simulink model "Scenario_2_v2"  (R2020b)
settings: Solver=ode1  StartTime=0.0  StopTime=10  FixedStep=Ts  MaxStep=Ts*2  MinStep=Ts/5  RelTol=1e-3
values from neighbouring files (symbols this model uses):
  c0 = c0_zeb    (= 6.57988e-09)    [Scenario_17_parameters_v2.m]    (also in Scenario_1_parameters_v2.m; Scenario_2_parameters_v2.m; Scenario_3_parameters_v2.m)
  c1 = c1_zeb    (= 9.15905e-09)    [Scenario_17_parameters_v2.m]    (also in Scenario_1_parameters_v2.m; Scenario_2_parameters_v2.m; Scenario_3_parameters_v2.m)
  fg = 50    [Scenario_17_parameters_v2.m]    (also in Scenario_1_parameters_v2.m; Scenario_2_parameters_v2.m; Scenario_3_parameters_v2.m)
  G1gen = 0.4692    [Scenario_17_parameters_v2.m]    (also in Scenario_1_parameters_v2.m = 0.1; Scenario_2_parameters_v2.m = 0.298581; Scenario_3_parameters_v2.m = 0.65)
  G2gen = 0.80    (= 0.8)    [Scenario_1_parameters_v2.m]    (also in Scenario_2_parameters_v2.m = 0.7; Scenario_3_parameters_v2.m = 0.4)
  G3gen = 0.85    [Scenario_1_parameters_v2.m]    (also in Scenario_2_parameters_v2.m = 0.9; Scenario_3_parameters_v2.m = 0.6)
  G4sgen = 0.8186    [Scenario_2_parameters_v2.m]
  G5gen = 0.75    [Scenario_17_parameters_v2.m]    (also in Scenario_1_parameters_v2.m = 0.8; Scenario_2_parameters_v2.m = 0.8; Scenario_3_parameters_v2.m = 0.705)
  G6gen = 0.90    (= 0.9)    [Scenario_17_parameters_v2.m]    (also in Scenario_1_parameters_v2.m; Scenario_2_parameters_v2.m = 0.81797; Scenario_3_parameters_v2.m = 0.45)
  G6sgen = 0.7    [Scenario_2_parameters_v2.m]
  G7gen = 0.20    (= 0.2)    [Scenario_17_parameters_v2.m]    (also in Scenario_1_parameters_v2.m = 0.5227; Scenario_2_parameters_v2.m = 0.5098; Scenario_3_parameters_v2.m = 0.4)
  Iovc = 1.2    [Scenario_17_parameters_v2.m]    (also in Scenario_1_parameters_v2.m; Scenario_2_parameters_v2.m; Scenario_3_parameters_v2.m)
  l0 = l0_zeb    (= 0.00368)    [Scenario_17_parameters_v2.m]    (also in Scenario_1_parameters_v2.m; Scenario_2_parameters_v2.m; Scenario_3_parameters_v2.m)
  l1 = l1_zeb    (= 0.00128)    [Scenario_17_parameters_v2.m]    (also in Scenario_1_parameters_v2.m; Scenario_2_parameters_v2.m; Scenario_3_parameters_v2.m)
  L3dem = 0.30    (= 0.3)    [Scenario_17_parameters_v2.m]    (also in Scenario_1_parameters_v2.m = 0.1; Scenario_2_parameters_v2.m = 0.1; Scenario_3_parameters_v2.m = 0.2)
  L4dem = 0.30    (= 0.3)    [Scenario_1_parameters_v2.m]    (also in Scenario_2_parameters_v2.m)
  L5dem = 0.25    [Scenario_17_parameters_v2.m]    (also in Scenario_1_parameters_v2.m = 0.35; Scenario_2_parameters_v2.m = 0.35; Scenario_3_parameters_v2.m = 0.1)
  L6dem = 0.15    [Scenario_1_parameters_v2.m]    (also in Scenario_2_parameters_v2.m; Scenario_3_parameters_v2.m = 0.1)
  L7dem = 0.10    (= 0.1)    [Scenario_1_parameters_v2.m]    (also in Scenario_2_parameters_v2.m; Scenario_3_parameters_v2.m = 0.2)
  Pr = Sr*PF    (= 1600500000)    [Scenario_17_parameters_v2.m]    (also in Scenario_1_parameters_v2.m = 1472500000; Scenario_2_parameters_v2.m = 1805000000; Scenario_3_parameters_v2.m = 12740000000)
  Qr = sqrt(Sr^2 - Pr^2)    [Scenario_17_parameters_v2.m]    (also in Scenario_1_parameters_v2.m; Scenario_2_parameters_v2.m; Scenario_3_parameters_v2.m)
  r0 = r0_zeb    (= 0.39362)    [Scenario_17_parameters_v2.m]    (also in Scenario_1_parameters_v2.m; Scenario_2_parameters_v2.m; Scenario_3_parameters_v2.m)
  r1 = r1_zeb    (= 0.06862)    [Scenario_17_parameters_v2.m]    (also in Scenario_1_parameters_v2.m; Scenario_2_parameters_v2.m; Scenario_3_parameters_v2.m)
  Rtpu = Xtpu/40    (= 0.0025)    [Scenario_17_parameters_v2.m]    (also in Scenario_1_parameters_v2.m = 0.00375; Scenario_2_parameters_v2.m = 0.00375; Scenario_3_parameters_v2.m)
  S1non = 700e6    (= 700000000)    [Scenario_17_parameters_v2.m]    (also in Scenario_1_parameters_v2.m = 400000000; Scenario_2_parameters_v2.m = 400000000; Scenario_3_parameters_v2.m = 1000000000)
  S2non = 300e6    (= 300000000)    [Scenario_1_parameters_v2.m]    (also in Scenario_2_parameters_v2.m; Scenario_3_parameters_v2.m = 3000000000)
  S3non = 200e6    (= 200000000)    [Scenario_1_parameters_v2.m]    (also in Scenario_2_parameters_v2.m; Scenario_3_parameters_v2.m = 1000000000)
  S4snon = 200e6    (= 200000000)    [Scenario_2_parameters_v2.m]
  S5non = 400e6    (= 400000000)    [Scenario_17_parameters_v2.m]    (also in Scenario_1_parameters_v2.m = 500000000; Scenario_2_parameters_v2.m = 500000000; Scenario_3_parameters_v2.m = 2000000000)
  S6non = 150e6    (= 150000000)    [Scenario_17_parameters_v2.m]    (also in Scenario_1_parameters_v2.m = 400000000; Scenario_2_parameters_v2.m = 400000000; Scenario_3_parameters_v2.m = 3000000000)
  S6snon = 200e6    (= 200000000)    [Scenario_2_parameters_v2.m]
  S7non = 1500e6    (= 1500000000)    [Scenario_17_parameters_v2.m]    (also in Scenario_1_parameters_v2.m = 200000000; Scenario_2_parameters_v2.m = 200000000; Scenario_3_parameters_v2.m = 4000000000)
  tonvsc = 0    [Scenario_17_parameters_v2.m]    (also in Scenario_1_parameters_v2.m; Scenario_2_parameters_v2.m; Scenario_3_parameters_v2.m = 0.0001)
  Ts = 50e-6    (= 5e-05)    [Scenario_17_parameters_v2.m]    (also in Scenario_1_parameters_v2.m = 0.0002; Scenario_2_parameters_v2.m = 2e-05; Scenario_3_parameters_v2.m = 0.0001)
  Vhv = 220e3    (= 220000)    [Scenario_17_parameters_v2.m]    (also in Scenario_1_parameters_v2.m; Scenario_2_parameters_v2.m; Scenario_3_parameters_v2.m)
  Vmv = 22e3    (= 22000)    [Scenario_17_parameters_v2.m]    (also in Scenario_1_parameters_v2.m; Scenario_2_parameters_v2.m; Scenario_3_parameters_v2.m)
  w_pll = 2*pi*80    (= 502.654824574)    [Scenario_17_parameters_v2.m]    (also in Scenario_1_parameters_v2.m; Scenario_2_parameters_v2.m; Scenario_3_parameters_v2.m)
  wc1 = wsw1/10    (= 848.230016469)    [Scenario_17_parameters_v2.m]    (also in Scenario_1_parameters_v2.m; Scenario_2_parameters_v2.m; Scenario_3_parameters_v2.m)
  wdc1 = wc1/10    (= 84.8230016469)    [Scenario_17_parameters_v2.m]    (also in Scenario_1_parameters_v2.m; Scenario_2_parameters_v2.m; Scenario_3_parameters_v2.m)
  wpq1 = wc1/10    (= 84.8230016469)    [Scenario_17_parameters_v2.m]    (also in Scenario_1_parameters_v2.m; Scenario_2_parameters_v2.m; Scenario_3_parameters_v2.m)
  wsw1 = ksw1*2*pi*fg    (= 8482.30016469)    [Scenario_17_parameters_v2.m]    (also in Scenario_1_parameters_v2.m; Scenario_2_parameters_v2.m; Scenario_3_parameters_v2.m)
  Xtpu = 0.10    (= 0.1)    [Scenario_17_parameters_v2.m]    (also in Scenario_1_parameters_v2.m = 0.15; Scenario_2_parameters_v2.m = 0.15; Scenario_3_parameters_v2.m)
undefined symbols (not defined in the file or in its folder): D11, Delta, Newton, Raphson
libraries: powerlib x214, simulink_extras x133, powerlib_meascontrol x102, pid_lib x48, simulink x32, eeTransforms x24, spsFirstOrderFilterLib x16, eePwmGeneratorTwoLevel x4
(part 18 of 19)

== system Scenario_2_v2/G6/VSC v2/VSC Control/Modulation/EMT Switching/Corrects delay1 ==
  Clock : Clock
  Filter delay : Constant  Commented=on  Value=tfilt
  Filter delay1 : Constant  Commented=on  Value=1/wsw1
  Gain : Gain  Gain=-2*pi*fg
  Memory : Memory
  Sum : Sum  Inputs=|+-
  Sum1 : Sum  Inputs=+++
  Sum2 : Sum  Inputs=|++
  Transformer connection : Constant  Value=pi/6
  dphi : Outport
  wires:
  Filter delay1/1 -> Sum1/1  "Tf"
  Filter delay/1 -> Sum1/3  "Tf"
  Sum/1 -> Sum1/2  "Ts"
  Clock/1 -> Memory/1, Sum/1
  Memory/1 -> Sum/2
  Sum1/1 -> Gain/1  "Td"
  Gain/1 -> Sum2/1
  Transformer connection/1 -> Sum2/2  "Tf"
  Sum2/1 -> dphi/1

== system Scenario_2_v2/G6/VSC v2/VSC Control/Modulation/Phasor I and Phasor PQ/Inverse Park Transform (Phasor) ==
  note: Transforming from real domain to complex domain
  note: In time domain, all variables are real.
      | In phasor domain, they are complex.
      | In phasor domain, what is seen as a variation in real domain is actually an angular displacement
      | As we know that the system is balanced, d and q have the same magnitude and are shifted 90 degrees
      | Thus, having the real parts and knowing that they are shifter 90 degrees, we can recover the complex part
  dq0 : Inport
  theta : Inport  Port=2
  Complex to Magnitude-Angle : ComplexToMagnitudeAngle  Commented=on
  Constant : Constant  Commented=on  Value=exp(-1i*2*pi/3)
  Constant1 : Constant  Commented=on  Value=exp(-1i*4*pi/3)
  Constant2 : Constant  Value=0
  Demux : Demux  Outputs=2
  Demux1 : Demux  Commented=on  Outputs=3
  Exp : Math  OutputSignalType=complex  SaturateOnIntegerOverflow=on
  Exp1 : Math  Commented=on  OutputSignalType=complex  SaturateOnIntegerOverflow=on
  First-Order Filter1 : spsFirstOrderFilterLib/First-Order Filter  Commented=on  FilterType=Lowpass  Tc=100e-6  Ts=0  Initialize=off  Vac_Init=[0, 0, 60]  Vdc_Init=0  PlotResponse=off  FreqRange="[0,  200,  1]"
  First-Order Filter2 : spsFirstOrderFilterLib/First-Order Filter  Commented=on  FilterType=Lowpass  Tc=100e-6  Ts=0  Initialize=off  Vac_Init=[0, 0, 60]  Vdc_Init=0  PlotResponse=off  FreqRange="[0,  200,  1]"
  Gain : Gain  Commented=on  Gain=exp(-1i*2*pi/3)
  Gain1 : Gain  Gain=1/2
  Gain2 : Gain  Gain=sqrt(3)
  Gain3 : Gain  Gain=1/2
  Gain4 : Gain  Gain=sqrt(3)
  Gain5 : Gain  Gain=1i
  Gain6 : Gain  Gain=-1
  Gain7 : Gain  Commented=on  Gain=1i
  Gain8 : Gain  Commented=on  Gain=exp(-1i*4*pi/3)
  Magnitude-Angle to Complex : MagnitudeAngleToComplex  Commented=on
  Mux : Mux  Commented=on  Inputs=3
  Mux2 : Mux  Inputs=3
  Product : Product
  Product1 : Product  Commented=on
  Real-Imag to Complex : RealImagToComplex
  Real-Imag to Complex1 : RealImagToComplex
  Sum : Sum  Inputs=|++
  Sum1 : Sum  Inputs=-|-
  Sum2 : Sum  Inputs=-|+
  Terminator : Terminator  Commented=on
  Terminator1 : Terminator  Commented=on
  abc : Outport  VectorParamsAs1DForOutWhenUnconnected=off
  wires:
  ? -> Demux1/1
  Demux1/3 -> Terminator1/1
  Magnitude-Angle to Complex/1 -> Gain/1, Mux/1, Gain8/1
  Gain/1 -> Mux/2
  Complex to Magnitude-Angle/1 -> First-Order Filter1/1
  Demux1/1 -> Complex to Magnitude-Angle/1
  Mux/1 -> ?
  Gain8/1 -> Mux/3
  Demux1/2 -> Terminator/1
  Complex to Magnitude-Angle/2 -> First-Order Filter2/1
  First-Order Filter2/1 -> Magnitude-Angle to Complex/2
  First-Order Filter1/1 -> Magnitude-Angle to Complex/1
  Sum/1 -> abc/1
  Constant2/1 -> [x0]
  Exp1/1 -> Product1/2
  Gain7/1 -> Exp1/1
  Gain6/1 -> Real-Imag to Complex1/2
  [xdr] -> Gain6/1
  [xqr] -> Real-Imag to Complex/2
  [xqr] -> Real-Imag to Complex1/1
  Real-Imag to Complex1/1 -> [xq]
  [xdr] -> Real-Imag to Complex/1
  Real-Imag to Complex/1 -> [xd]
  Gain3/1 -> Mux2/3
  Gain1/1 -> Mux2/2
  Sum2/1 -> Gain3/1
  [xd] -> Gain4/1
  [xq] -> Sum2/1
  Gain4/1 -> Sum2/2
  Gain2/1 -> Sum1/2
  [xd] -> Gain2/1
  [xq] -> Sum1/1
  Sum1/1 -> Gain1/1
  [xq] -> Mux2/1
  theta/1 -> Gain5/1
  Gain5/1 -> Exp/1
  Mux2/1 -> Product/1
  Exp/1 -> Product/2
  Product/1 -> Sum/1
  [x0] -> Sum/2
  Demux/2 -> [xqr]
  Demux/1 -> [xdr]
  dq0/1 -> Demux/1

== system Scenario_2_v2/G6/VSC v2/VSC Control/Modulation/Phasor I and Phasor PQ/Subsystem ==
  note: Symmetrical components to ABC
  012 : Inport
  Gain1 : Gain  Gain=[1 a a2]  SaturateOnIntegerOverflow=on  OutDataTypeStr=Inherit: Same as input  ParamDataTypeStr=Inherit: Same as input
  Gain2 : Gain  Gain=[1 a2 a]  SaturateOnIntegerOverflow=on  OutDataTypeStr=Inherit: Same as input  ParamDataTypeStr=Inherit: Same as input
  Mux : Mux  Inputs=3
  Sum : Sum  Inputs=1  InputSameDT=on  SaturateOnIntegerOverflow=on  OutDataTypeStr=Inherit: Same as first input
  Sum1 : Sum  Inputs=1  InputSameDT=on  SaturateOnIntegerOverflow=on  OutDataTypeStr=Inherit: Same as first input
  Sum2 : Sum  Inputs=1  InputSameDT=on  SaturateOnIntegerOverflow=on  OutDataTypeStr=Inherit: Same as first input
  abc : Outport
  wires:
  Mux/1 -> abc/1
  Sum2/1 -> Mux/1
  Sum/1 -> Mux/2
  Sum1/1 -> Mux/3
  Gain1/1 -> Sum1/1
  012/1 -> Gain2/1, Sum2/1, Gain1/1
  Gain2/1 -> Sum/1

== system Scenario_2_v2/G6/VSC v2/VSC Control/Modulation/Phasor Quasi-EMT/Corrects delay ==
  Clock : Clock
  Gain : Gain  Gain=(2*pi*fg)
  Memory : Memory
  Sum : Sum  Inputs=|+-
  Sum2 : Sum  Inputs=|++
  Transformer connection : Constant  Commented=on  Value=pi/6
  dphi : Outport
  wires:
  Clock/1 -> Memory/1, Sum/1
  Memory/1 -> Sum/2
  Sum/1 -> Gain/1  "Ts"
  Transformer connection/1 -> Sum2/2  "Tf"
  Gain/1 -> Sum2/1
  Sum2/1 -> dphi/1

== system Scenario_2_v2/G6/VSC v2/VSC Control/Modulation/Phasor Quasi-EMT/Corrects delay2 ==
  Clock : Clock
  Gain : Gain  Gain=(2*pi*fg)
  Memory : Memory
  Sum : Sum  Inputs=|+-
  Sum2 : Sum  Inputs=|++
  Transformer connection : Constant  Commented=on  Value=pi/6
  dphi : Outport
  wires:
  Clock/1 -> Memory/1, Sum/1
  Memory/1 -> Sum/2
  Sum/1 -> Gain/1  "Ts"
  Transformer connection/1 -> Sum2/2  "Tf"
  Gain/1 -> Sum2/1
  Sum2/1 -> dphi/1

== system Scenario_2_v2/G6/VSC v2/VSC Control/Modulation/Phasor Quasi-EMT/Inverse Park Transform (Phasor) ==
  note: In time domain, all variables are real.
      | In phasor domain, they are complex.
      | In phasor domain, what is seen as a variation in real domain is actually an angular displacement
      | As we know that the system is balanced, d and q have the same magnitude and are shifted 90 degrees
      | Thus, having the real parts and knowing that they are shifter 90 degrees, we can recover the complex part
  note: Transforming from real domain to complex domain
  dq0 : Inport
  theta : Inport  Port=2
  Complex to Magnitude-Angle : ComplexToMagnitudeAngle  Commented=on
  Constant : Constant  Commented=on  Value=exp(-1i*2*pi/3)
  Constant1 : Constant  Commented=on  Value=exp(-1i*4*pi/3)
  Constant2 : Constant  Value=0
  Demux : Demux  Outputs=2
  Demux1 : Demux  Commented=on  Outputs=3
  Exp : Math  OutputSignalType=complex  SaturateOnIntegerOverflow=on
  Exp1 : Math  Commented=on  OutputSignalType=complex  SaturateOnIntegerOverflow=on
  First-Order Filter1 : spsFirstOrderFilterLib/First-Order Filter  Commented=on  FilterType=Lowpass  Tc=100e-6  Ts=0  Initialize=off  Vac_Init=[0, 0, 60]  Vdc_Init=0  PlotResponse=off  FreqRange="[0,  200,  1]"
  First-Order Filter2 : spsFirstOrderFilterLib/First-Order Filter  Commented=on  FilterType=Lowpass  Tc=100e-6  Ts=0  Initialize=off  Vac_Init=[0, 0, 60]  Vdc_Init=0  PlotResponse=off  FreqRange="[0,  200,  1]"
  Gain : Gain  Commented=on  Gain=exp(-1i*2*pi/3)
  Gain1 : Gain  Gain=1/2
  Gain2 : Gain  Gain=sqrt(3)
  Gain3 : Gain  Gain=1/2
  Gain4 : Gain  Gain=sqrt(3)
  Gain5 : Gain  Gain=1i
  Gain6 : Gain  Gain=-1
  Gain7 : Gain  Commented=on  Gain=1i
  Gain8 : Gain  Commented=on  Gain=exp(-1i*4*pi/3)
  Magnitude-Angle to Complex : MagnitudeAngleToComplex  Commented=on
  Mux : Mux  Commented=on  Inputs=3
  Mux2 : Mux  Inputs=3
  Product : Product
  Product1 : Product  Commented=on
  Real-Imag to Complex : RealImagToComplex
  Real-Imag to Complex1 : RealImagToComplex
  Sum : Sum  Inputs=|++
  Sum1 : Sum  Inputs=-|-
  Sum2 : Sum  Inputs=-|+
  Terminator : Terminator  Commented=on
  Terminator1 : Terminator  Commented=on
  abc : Outport  VectorParamsAs1DForOutWhenUnconnected=off
  wires:
  dq0/1 -> Demux/1
  Demux/1 -> [xdr]
  Demux/2 -> [xqr]
  [x0] -> Sum/2
  Product/1 -> Sum/1
  Exp/1 -> Product/2
  Mux2/1 -> Product/1
  Gain5/1 -> Exp/1
  theta/1 -> Gain5/1
  [xq] -> Mux2/1
  Sum1/1 -> Gain1/1
  [xq] -> Sum1/1
  [xd] -> Gain2/1
  Gain2/1 -> Sum1/2
  Gain4/1 -> Sum2/2
  [xq] -> Sum2/1
  [xd] -> Gain4/1
  Sum2/1 -> Gain3/1
  Gain1/1 -> Mux2/2
  Gain3/1 -> Mux2/3
  Real-Imag to Complex/1 -> [xd]
  [xdr] -> Real-Imag to Complex/1
  Real-Imag to Complex1/1 -> [xq]
  [xqr] -> Real-Imag to Complex1/1
  [xqr] -> Real-Imag to Complex/2
  [xdr] -> Gain6/1
  Gain6/1 -> Real-Imag to Complex1/2
  Gain7/1 -> Exp1/1
  Exp1/1 -> Product1/2
  Constant2/1 -> [x0]
  Sum/1 -> abc/1
  First-Order Filter1/1 -> Magnitude-Angle to Complex/1
  First-Order Filter2/1 -> Magnitude-Angle to Complex/2
  Complex to Magnitude-Angle/2 -> First-Order Filter2/1
  Demux1/2 -> Terminator/1
  Gain8/1 -> Mux/3
  Mux/1 -> ?
  Demux1/1 -> Complex to Magnitude-Angle/1
  Complex to Magnitude-Angle/1 -> First-Order Filter1/1
  Gain/1 -> Mux/2
  Magnitude-Angle to Complex/1 -> Gain8/1, Mux/1, Gain/1
  Demux1/3 -> Terminator1/1
  ? -> Demux1/1

== system Scenario_2_v2/G6/VSC v2/VSC Control/Modulation/Phasor Quasi-EMT/Subsystem ==
  note: Symmetrical components to ABC
  012 : Inport
  Gain1 : Gain  Gain=[1 a a2]  SaturateOnIntegerOverflow=on  OutDataTypeStr=Inherit: Same as input  ParamDataTypeStr=Inherit: Same as input
  Gain2 : Gain  Gain=[1 a2 a]  SaturateOnIntegerOverflow=on  OutDataTypeStr=Inherit: Same as input  ParamDataTypeStr=Inherit: Same as input
  Mux : Mux  Inputs=3
  Sum : Sum  Inputs=1  InputSameDT=on  SaturateOnIntegerOverflow=on  OutDataTypeStr=Inherit: Same as first input
  Sum1 : Sum  Inputs=1  InputSameDT=on  SaturateOnIntegerOverflow=on  OutDataTypeStr=Inherit: Same as first input
  Sum2 : Sum  Inputs=1  InputSameDT=on  SaturateOnIntegerOverflow=on  OutDataTypeStr=Inherit: Same as first input
  abc : Outport
  wires:
  Gain2/1 -> Sum/1
  012/1 -> Gain1/1, Sum2/1, Gain2/1
  Gain1/1 -> Sum1/1
  Sum1/1 -> Mux/3
  Sum/1 -> Mux/2
  Sum2/1 -> Mux/1
  Mux/1 -> abc/1

== system Scenario_2_v2/G6/VSC v2/VSC Control/Modulation/Phasor Quasi-EMT/V to I RL (+seq) ==
  note: d-q axis model of a 3-phase series R-L branch
  note: Using Laplace transform:
  note: Iq = (Vq1 - Vq2 - w*L*Id)/(R + s*L)
  note: Id = (Vd1 - Vd2 + w*L*Iq)/(R + s*L)
  note: V2
  note: ==========================================================================================
  note: V1
  note: Vq1 - Vq2 = [ R * Iq ] + [ L* w * Id ] + [ L * d/dt (Iq) ]
  note: where w = 2*pi*f
  note: I --->
  note: o--------| R |---| L |-------o
  note: Vd1 - Vd2 = [ R * Id ] - [ L* w * Iq ] + [ L * d/dt (Id) ]
  note: This subsystem converts the VSC output voltage in a current signal through an RL element
  Vdq1 : Inport
  Vdq2 : Inport  Port=2
  Cartesian to Polar : simulink_extras/Transformations/Cartesian to Polar
  Delay : Delay  DelayLength=1
  Demux : Demux  Outputs=2
  IC : InitialCondition  Value=Tcd
  IC1 : InitialCondition  Value=Tcq
  Mux : Mux  Inputs=2
  Polar to Cartesian : simulink_extras/Transformations/Polar to Cartesian
      settings: SourceProductBaseCode=SL
  R_choke1 : Gain  Gain=w*L  SaturateOnIntegerOverflow=on  OutDataTypeStr=Inherit: Same as input  ParamDataTypeStr=Inherit: Same as input
  R_choke2 : Gain  Gain=[1 -1]  SaturateOnIntegerOverflow=on  OutDataTypeStr=Inherit: Same as input  ParamDataTypeStr=Inherit: Same as input
  Saturation : Saturate  UpperLimit=Imax  LowerLimit=0
  Selector : Selector  InputPortWidth=2  IndexOptions=Index vector (dialog)  Indices=[2 1]  OutputSizes=1
  Sum : Sum  Inputs=+-+  SaturateOnIntegerOverflow=on
  Transfer Fcn (with initial outputs) : simulink_extras/Additional Linear/Transfer Fcn (with initial outputs)  N=[1]  D=[L R]  Y0=Icd  U0=Tcd
  Transfer Fcn (with initial outputs)1 : simulink_extras/Additional Linear/Transfer Fcn (with initial outputs)  N=[1]  D=[L R]  Y0=Icq  U0=Tcq
  idIq : Outport  VectorParamsAs1DForOutWhenUnconnected=off
  wires:
  Selector/1 -> R_choke1/1
  Vdq1/1 -> Sum/1
  R_choke1/1 -> R_choke2/1
  Demux/1 -> IC/1
  Demux/2 -> IC1/1
  Polar to Cartesian/1 -> Mux/1
  Polar to Cartesian/2 -> Mux/2
  Cartesian to Polar/2 -> Polar to Cartesian/2
  R_choke2/1 -> Sum/3
  Transfer Fcn (with initial outputs)/1 -> Cartesian to Polar/1
  Transfer Fcn (with initial outputs)1/1 -> Cartesian to Polar/2
  Vdq2/1 -> Sum/2
  Cartesian to Polar/1 -> Saturation/1
  Saturation/1 -> Polar to Cartesian/1
  Delay/1 -> Selector/1
  IC/1 -> Transfer Fcn (with initial outputs)/1
  IC1/1 -> Transfer Fcn (with initial outputs)1/1
  Mux/1 -> Delay/1, idIq/1
  Sum/1 -> Demux/1

== system Scenario_2_v2/G6/VSC v2/VSC Control/Modulation/Phasor Quasi-EMT/V to I RL (- seq) ==
  note: d-q axis model of a 3-phase series R-L branch
  note: Using Laplace transform:
  note: Iq = (Vq1 - Vq2 - w*L*Id)/(R + s*L)
  note: Id = (Vd1 - Vd2 + w*L*Iq)/(R + s*L)
  note: V2
  note: ==========================================================================================
  note: V1
  note: Vq1 - Vq2 = [ R * Iq ] + [ L* w * Id ] + [ L * d/dt (Iq) ]
  note: where w = 2*pi*f
  note: I --->
  note: o--------| R |---| L |-------o
  note: Vd1 - Vd2 = [ R * Id ] - [ L* w * Iq ] + [ L * d/dt (Id) ]
  note: This subsystem converts the VSC output voltage in a current signal through an RL element
  Vdq1 : Inport
  Vdq2 : Inport  Port=2
  Cartesian to Polar : simulink_extras/Transformations/Cartesian to Polar
  Delay : Delay  DelayLength=1
  Demux : Demux  Outputs=2
  Mux : Mux  Inputs=2
  Polar to Cartesian : simulink_extras/Transformations/Polar to Cartesian
      settings: SourceProductBaseCode=SL
  R_choke1 : Gain  Gain=w*L  SaturateOnIntegerOverflow=on  OutDataTypeStr=Inherit: Same as input  ParamDataTypeStr=Inherit: Same as input
  R_choke2 : Gain  Gain=[-1 1]  SaturateOnIntegerOverflow=on  OutDataTypeStr=Inherit: Same as input  ParamDataTypeStr=Inherit: Same as input
  Saturation : Saturate  UpperLimit=Imax  LowerLimit=0
  Selector : Selector  InputPortWidth=2  IndexOptions=Index vector (dialog)  Indices=[2 1]  OutputSizes=1
  Sum : Sum  Inputs=+-+  SaturateOnIntegerOverflow=on
  Transfer Fcn (with initial outputs) : simulink_extras/Additional Linear/Transfer Fcn (with initial outputs)  N=[1]  D=[L R]  Y0=0  U0=0
  Transfer Fcn (with initial outputs)1 : simulink_extras/Additional Linear/Transfer Fcn (with initial outputs)  N=[1]  D=[L R]  Y0=0  U0=0
  idIq : Outport  VectorParamsAs1DForOutWhenUnconnected=off
  wires:
  Selector/1 -> R_choke1/1
  Vdq1/1 -> Sum/1
  R_choke1/1 -> R_choke2/1
  Sum/1 -> Demux/1
  Demux/1 -> Transfer Fcn (with initial outputs)/1
  Demux/2 -> Transfer Fcn (with initial outputs)1/1
  Polar to Cartesian/1 -> Mux/1
  Polar to Cartesian/2 -> Mux/2
  Cartesian to Polar/2 -> Polar to Cartesian/2
  Mux/1 -> Delay/1, idIq/1
  R_choke2/1 -> Sum/3
  Transfer Fcn (with initial outputs)/1 -> Cartesian to Polar/1
  Transfer Fcn (with initial outputs)1/1 -> Cartesian to Polar/2
  Vdq2/1 -> Sum/2
  Cartesian to Polar/1 -> Saturation/1
  Saturation/1 -> Polar to Cartesian/1
  Delay/1 -> Selector/1

== system Scenario_2_v2/G2/VSC v2/VSC Control/Control loops/Phasor I 1st/Outer-loop/Power calculation ==
  note: AC power calculation using symmetrical components in dq axis
  note: Pavgp = 3/2*(vqp*iqp + vdp*idp) and Qavgp = 3/2*(vqp*idp-vdp*iqp)
  note: P = Pavg + Pc2*cos(2wt) + Ps2*sin(2wt) ---> Pavg = Pavgp + Pavgn
  note: Q = Qavg + Qc2*cos(2wt) + Qs2*sin(2wt) ---> Qavg = Qavgp + Qavgn
  note: Pavgn = 3/2*(vqn*iqn + vdn*idn) and Qavgn = 3/2*(vqn*idn-vdn*iqn)
  vq+ : Inport
  vd+ : Inport  Port=2
  iq+ : Inport  Port=3
  id+ : Inport  Port=4
  vq- : Inport  Port=5
  vd- : Inport  Port=6
  iq- : Inport  Port=7
  id- : Inport  Port=8
  Gain : Gain  Gain=3/2
  Gain1 : Gain  Gain=3/2
  Gain2 : Gain  Gain=-1
  Gain3 : Gain  Gain=-1
  Gain4 : Gain  Gain=negseq_en
  Mux{,1..3} (4 alike) : Mux  Inputs=2
  Product{,1..3} (4 alike) : Product
  Sum1 : Sum
  Sum2 : Sum
  Sum8 : Sum
  PQ : Outport
  wires:
  Sum8/1 -> Gain/1
  Gain2/1 -> Mux2/2
  Mux2/1 -> Product2/2
  Product2/1 -> Sum8/2
  Mux/1 -> Product/2
  Product/1 -> Sum8/1
  iq+/1 -> [iqp]
  [iqp] -> Gain2/1, Mux/1
  id+/1 -> [idp]
  [idp] -> Mux2/1, Mux/2
  vq+/1 -> [vqp]
  [vqp] -> Product/1
  vd+/1 -> [vdp]
  [vdp] -> Product2/1
  Gain/1 -> Sum1/1
  Sum1/1 -> PQ/1
  Gain3/1 -> Mux3/2
  Mux1/1 -> Product1/2
  Product3/1 -> Sum2/2
  Product1/1 -> Sum2/1
  [vdn] -> Product3/1
  Mux3/1 -> Product3/2
  [vqn] -> Product1/1
  Sum2/1 -> Gain1/1
  [iqn] -> Gain3/1, Mux1/1
  [idn] -> Mux3/1, Mux1/2
  vq-/1 -> [vqn]
  vd-/1 -> [vdn]
  iq-/1 -> [iqn]
  id-/1 -> [idn]
  Gain1/1 -> Gain4/1
  Gain4/1 -> Sum1/2

== system Scenario_2_v2/G2/VSC v2/VSC Control/Control loops/Phasor I ref/Outer-loop/Power calculation ==
  note: AC power calculation using symmetrical components in dq axis
  note: Pavgp = 3/2*(vqp*iqp + vdp*idp) and Qavgp = 3/2*(vqp*idp-vdp*iqp)
  note: P = Pavg + Pc2*cos(2wt) + Ps2*sin(2wt) ---> Pavg = Pavgp + Pavgn
  note: Q = Qavg + Qc2*cos(2wt) + Qs2*sin(2wt) ---> Qavg = Qavgp + Qavgn
  note: Pavgn = 3/2*(vqn*iqn + vdn*idn) and Qavgn = 3/2*(vqn*idn-vdn*iqn)
  vq+ : Inport
  vd+ : Inport  Port=2
  iq+ : Inport  Port=3
  id+ : Inport  Port=4
  vq- : Inport  Port=5
  vd- : Inport  Port=6
  iq- : Inport  Port=7
  id- : Inport  Port=8
  Gain : Gain  Gain=3/2
  Gain1 : Gain  Gain=3/2
  Gain2 : Gain  Gain=-1
  Gain3 : Gain  Gain=-1
  Gain4 : Gain  Gain=negseq_en
  Mux{,1..3} (4 alike) : Mux  Inputs=2
  Product{,1..3} (4 alike) : Product
  Sum1 : Sum
  Sum2 : Sum
  Sum8 : Sum
  PQ : Outport
  wires:
  Sum8/1 -> Gain/1
  Gain2/1 -> Mux2/2
  Mux2/1 -> Product2/2
  Product2/1 -> Sum8/2
  Mux/1 -> Product/2
  Product/1 -> Sum8/1
  iq+/1 -> [iqp]
  [iqp] -> Gain2/1, Mux/1
  id+/1 -> [idp]
  [idp] -> Mux2/1, Mux/2
  vq+/1 -> [vqp]
  [vqp] -> Product/1
  vd+/1 -> [vdp]
  [vdp] -> Product2/1
  Gain/1 -> Sum1/1
  Sum1/1 -> PQ/1
  Gain3/1 -> Mux3/2
  Mux1/1 -> Product1/2
  Product3/1 -> Sum2/2
  Product1/1 -> Sum2/1
  [vdn] -> Product3/1
  Mux3/1 -> Product3/2
  [vqn] -> Product1/1
  Sum2/1 -> Gain1/1
  [iqn] -> Gain3/1, Mux1/1
  [idn] -> Mux3/1, Mux1/2
  vq-/1 -> [vqn]
  vd-/1 -> [vdn]
  iq-/1 -> [iqn]
  id-/1 -> [idn]
  Gain1/1 -> Gain4/1
  Gain4/1 -> Sum1/2

== system Scenario_2_v2/G2/VSC v2/VSC Control/Control loops/Phasor PQ 1st/Outer-loop/Power calculation ==
  note: AC power calculation using symmetrical components in dq axis
  note: Pavgp = 3/2*(vqp*iqp + vdp*idp) and Qavgp = 3/2*(vqp*idp-vdp*iqp)
  note: P = Pavg + Pc2*cos(2wt) + Ps2*sin(2wt) ---> Pavg = Pavgp + Pavgn
  note: Q = Qavg + Qc2*cos(2wt) + Qs2*sin(2wt) ---> Qavg = Qavgp + Qavgn
  note: Pavgn = 3/2*(vqn*iqn + vdn*idn) and Qavgn = 3/2*(vqn*idn-vdn*iqn)
  vq+ : Inport
  vd+ : Inport  Port=2
  iq+ : Inport  Port=3
  id+ : Inport  Port=4
  vq- : Inport  Port=5
  vd- : Inport  Port=6
  iq- : Inport  Port=7
  id- : Inport  Port=8
  Gain : Gain  Gain=3/2
  Gain1 : Gain  Gain=3/2
  Gain2 : Gain  Gain=-1
  Gain3 : Gain  Gain=-1
  Gain4 : Gain  Gain=negseq_en
  Mux{,1..3} (4 alike) : Mux  Inputs=2
  Product{,1..3} (4 alike) : Product
  Sum1 : Sum
  Sum2 : Sum
  Sum8 : Sum
  PQ : Outport
  wires:
  Sum8/1 -> Gain/1
  Gain2/1 -> Mux2/2
  Mux2/1 -> Product2/2
  Product2/1 -> Sum8/2
  Mux/1 -> Product/2
  Product/1 -> Sum8/1
  iq+/1 -> [iqp]
  [iqp] -> Gain2/1, Mux/1
  id+/1 -> [idp]
  [idp] -> Mux2/1, Mux/2
  vq+/1 -> [vqp]
  [vqp] -> Product/1
  vd+/1 -> [vdp]
  [vdp] -> Product2/1
  Gain/1 -> Sum1/1
  Sum1/1 -> PQ/1
  Gain3/1 -> Mux3/2
  Mux1/1 -> Product1/2
  Product3/1 -> Sum2/2
  Product1/1 -> Sum2/1
  [vdn] -> Product3/1
  Mux3/1 -> Product3/2
  [vqn] -> Product1/1
  Sum2/1 -> Gain1/1
  [iqn] -> Gain3/1, Mux1/1
  [idn] -> Mux3/1, Mux1/2
  vq-/1 -> [vqn]
  vd-/1 -> [vdn]
  iq-/1 -> [iqn]
  id-/1 -> [idn]
  Gain1/1 -> Gain4/1
  Gain4/1 -> Sum1/2

== system Scenario_2_v2/G2/VSC v2/VSC Control/Control loops/SW, EMT AVG, Phasor Quasi-EMT/Outer-loop/Power calculation ==
  note: AC power calculation using symmetrical components in dq axis
  note: Pavgp = 3/2*(vqp*iqp + vdp*idp) and Qavgp = 3/2*(vqp*idp-vdp*iqp)
  note: P = Pavg + Pc2*cos(2wt) + Ps2*sin(2wt) ---> Pavg = Pavgp + Pavgn
  note: Q = Qavg + Qc2*cos(2wt) + Qs2*sin(2wt) ---> Qavg = Qavgp + Qavgn
  note: Pavgn = 3/2*(vqn*iqn + vdn*idn) and Qavgn = 3/2*(vqn*idn-vdn*iqn)
  vq+ : Inport
  vd+ : Inport  Port=2
  iq+ : Inport  Port=3
  id+ : Inport  Port=4
  vq- : Inport  Port=5
  vd- : Inport  Port=6
  iq- : Inport  Port=7
  id- : Inport  Port=8
  Gain : Gain  Gain=3/2
  Gain1 : Gain  Gain=3/2
  Gain2 : Gain  Gain=-1
  Gain3 : Gain  Gain=-1
  Gain4 : Gain  Gain=negseq_en
  Mux{,1..3} (4 alike) : Mux  Inputs=2
  Product{,1..3} (4 alike) : Product
  Sum1 : Sum
  Sum2 : Sum
  Sum8 : Sum
  PQ : Outport
  wires:
  Sum8/1 -> Gain/1
  Gain2/1 -> Mux2/2
  Mux2/1 -> Product2/2
  Product2/1 -> Sum8/2
  Mux/1 -> Product/2
  Product/1 -> Sum8/1
  iq+/1 -> [iqp]
  [iqp] -> Gain2/1, Mux/1
  id+/1 -> [idp]
  [idp] -> Mux2/1, Mux/2
  vq+/1 -> [vqp]
  [vqp] -> Product/1
  vd+/1 -> [vdp]
  [vdp] -> Product2/1
  Gain/1 -> Sum1/1
  Sum1/1 -> PQ/1
  Gain3/1 -> Mux3/2
  Mux1/1 -> Product1/2
  Product3/1 -> Sum2/2
  Product1/1 -> Sum2/1
  [vdn] -> Product3/1
  Mux3/1 -> Product3/2
  [vqn] -> Product1/1
  Sum2/1 -> Gain1/1
  [iqn] -> Gain3/1, Mux1/1
  [idn] -> Mux3/1, Mux1/2
  vq-/1 -> [vqn]
  vd-/1 -> [vdn]
  iq-/1 -> [iqn]
  id-/1 -> [idn]
  Gain1/1 -> Gain4/1
  Gain4/1 -> Sum1/2

== system Scenario_2_v2/G2/VSC v2/VSC Control/Control loops/SW, EMT AVG, Phasor Quasi-EMT/Outer-loop/Subsystem2 ==
  note: Hold initial variable value for a given time
  In1 : Inport
  Constant : Constant  Value=x0
  Constant1 : Constant
  Integrator : Integrator
  Switch : Switch  Threshold=Td
  Out1 : Outport
  wires:
  Integrator/1 -> Switch/2
  In1/1 -> Switch/1
  Switch/1 -> Out1/1
  Constant/1 -> Switch/3
  Constant1/1 -> Integrator/1

== system Scenario_2_v2/G2/VSC v2/VSC Control/Control loops/SW, EMT AVG, Phasor Quasi-EMT/Outer-loop/Subsystem3 ==
  note: Hold initial variable value for a given time
  In1 : Inport
  Constant : Constant  Value=x0
  Constant1 : Constant
  Integrator : Integrator
  Switch : Switch  Threshold=Td
  Out1 : Outport
  wires:
  Integrator/1 -> Switch/2
  In1/1 -> Switch/1
  Switch/1 -> Out1/1
  Constant/1 -> Switch/3
  Constant1/1 -> Integrator/1

== system Scenario_2_v2/G2/VSC v2/VSC Control/Measurements/EMT/PLL aligned with positive-sequence/Phase-sequence separation ==
  note: Phase-sequence separation based on
      | Delayed Signal Cancellation (DSC) method
  abc : Inport
  Theta : Inport  Port=2
  Complex to Real-Imag1 : ComplexToRealImag
  Complex to Real-Imag2 : ComplexToRealImag
  Complex to Real-Imag3 : ComplexToRealImag
  Constant : Constant  Value=negseq_en
  Demux3 : Demux  Outputs=3
  Exp2 : Math  OutputSignalType=complex  SaturateOnIntegerOverflow=on
  Exp3 : Math  OutputSignalType=complex  SaturateOnIntegerOverflow=on
  Gain1 : Gain  Gain=1/2
  Gain4 : Gain  Gain=-1i
  Gain5 : Gain  Gain=1i
  Gain6 : Gain  Gain=1/2
  Gain7 : Gain  Gain=1i
  NOT : Logic  Operator=NOT  IconShape=distinctive  AllPortsSameDT=off  OutDataTypeStr=boolean
  Product3 : Product
  Product4 : Product
  Real-Imag to Complex : RealImagToComplex
  Real-Imag to Complex1 : RealImagToComplex
  Sum1 : Sum  Inputs=|++
  Sum2 : Sum  Inputs=-+|
  Switch : Switch  Criteria=u2 ~= 0
  Terminator3 : Terminator
  Transport Delay2 : TransportDelay  DelayTime=1/4*(1/fg)  BufferSize=1024*4
  Transport Delay3 : TransportDelay  DelayTime=1/4*(1/fg)  BufferSize=1024*4
  abc to Alpha-Beta-Zero : powerlib_meascontrol/Transformations/abc to Alpha-Beta-Zero
  q+ : Outport
  d+ : Outport  Port=2
  q- : Outport  Port=3
  d- : Outport  Port=4
  wires:
  NOT/1 -> Switch/2
  Constant/1 -> NOT/1
  Switch/1 -> Product3/1
  Gain6/1 -> Switch/3
  Sum2/1 -> Gain1/1
  Transport Delay2/1 -> Real-Imag to Complex1/1
  Demux3/1 -> Real-Imag to Complex/1
  Complex to Real-Imag1/2 -> Transport Delay3/1
  Gain1/1 -> Product4/2
  Real-Imag to Complex/1 -> Complex to Real-Imag1/1, Sum2/2, Sum1/1, Switch/1
  Complex to Real-Imag3/1 -> d-/1
  Real-Imag to Complex1/1 -> Gain5/1
  Complex to Real-Imag1/1 -> Transport Delay2/1
  Transport Delay3/1 -> Real-Imag to Complex1/2
  Demux3/2 -> Real-Imag to Complex/2
  Product3/1 -> Complex to Real-Imag2/1
  Product4/1 -> Complex to Real-Imag3/1
  abc to Alpha-Beta-Zero/1 -> Demux3/1
  abc/1 -> abc to Alpha-Beta-Zero/1
  Exp3/1 -> Product4/1
  Complex to Real-Imag3/2 -> q-/1
  Complex to Real-Imag2/2 -> q+/1
  Demux3/3 -> Terminator3/1
  Sum1/1 -> Gain6/1
  Gain5/1 -> Sum2/1, Sum1/2
  Exp2/1 -> Product3/2
  Gain4/1 -> Exp2/1
  Theta/1 -> Gain4/1, Gain7/1
  Gain7/1 -> Exp3/1
  Complex to Real-Imag2/1 -> d+/1

== system Scenario_2_v2/G2/VSC v2/VSC Control/Measurements/EMT/PLL aligned with positive-sequence/Subsystem ==
  note: PI controller with reset port and initial conditions restored after reset or after maximum/minimum values are reached
  in : Inport
  Reset : Inport  Port=2
  Compare To Constant2 : simulink/Logic and Bit Operations/Compare To Constant  relop=~=  const=0  OutDataTypeStr=boolean
  Constant2 : Constant  Value=2*pi*fg
  Gain : Gain  Gain=kp_pll
  Gain1 : Gain  Gain=kp_pll/tau_pll
  Integrator Limited : Integrator  ExternalReset=level  InitialCondition=2*pi*fg  UpperSaturationLimit=10.1*2*pi*fg  LowerSaturationLimit=0.09*2*pi*fg  ShowSaturationPort=on
  Memory1 : Memory
  NOT : Logic  Operator=NOT  IconShape=distinctive  AllPortsSameDT=off  OutDataTypeStr=boolean
  OR2 : Logic  Operator=OR  IconShape=distinctive  AllPortsSameDT=off  OutDataTypeStr=boolean
  Product : Product
  Sum : Sum
  Switch1 : Switch
  w : Outport
  wires:
  Switch1/1 -> w/1
  Product/1 -> Gain1/1, Gain/1
  Gain1/1 -> Integrator Limited/1
  Integrator Limited/2 -> Compare To Constant2/1, Switch1/2
  Compare To Constant2/1 -> Memory1/1
  OR2/1 -> Integrator Limited/2, NOT/1
  Constant2/1 -> Switch1/3
  Memory1/1 -> OR2/1
  Reset/1 -> OR2/2
  Gain/1 -> Sum/1
  Integrator Limited/1 -> Sum/2
  Sum/1 -> Switch1/1
  in/1 -> Product/1
  NOT/1 -> Product/2

== system Scenario_2_v2/G3/VSC v2/VSC Control/Control loops/Phasor I 1st/Outer-loop/Power calculation ==
  note: AC power calculation using symmetrical components in dq axis
  note: Pavgp = 3/2*(vqp*iqp + vdp*idp) and Qavgp = 3/2*(vqp*idp-vdp*iqp)
  note: P = Pavg + Pc2*cos(2wt) + Ps2*sin(2wt) ---> Pavg = Pavgp + Pavgn
  note: Q = Qavg + Qc2*cos(2wt) + Qs2*sin(2wt) ---> Qavg = Qavgp + Qavgn
  note: Pavgn = 3/2*(vqn*iqn + vdn*idn) and Qavgn = 3/2*(vqn*idn-vdn*iqn)
  vq+ : Inport
  vd+ : Inport  Port=2
  iq+ : Inport  Port=3
  id+ : Inport  Port=4
  vq- : Inport  Port=5
  vd- : Inport  Port=6
  iq- : Inport  Port=7
  id- : Inport  Port=8
  Gain : Gain  Gain=3/2
  Gain1 : Gain  Gain=3/2
  Gain2 : Gain  Gain=-1
  Gain3 : Gain  Gain=-1
  Gain4 : Gain  Gain=negseq_en
  Mux{,1..3} (4 alike) : Mux  Inputs=2
  Product{,1..3} (4 alike) : Product
  Sum1 : Sum
  Sum2 : Sum
  Sum8 : Sum
  PQ : Outport
  wires:
  Sum8/1 -> Gain/1
  Gain2/1 -> Mux2/2
  Mux2/1 -> Product2/2
  Product2/1 -> Sum8/2
  Mux/1 -> Product/2
  Product/1 -> Sum8/1
  iq+/1 -> [iqp]
  [iqp] -> Gain2/1, Mux/1
  id+/1 -> [idp]
  [idp] -> Mux2/1, Mux/2
  vq+/1 -> [vqp]
  [vqp] -> Product/1
  vd+/1 -> [vdp]
  [vdp] -> Product2/1
  Gain/1 -> Sum1/1
  Sum1/1 -> PQ/1
  Gain3/1 -> Mux3/2
  Mux1/1 -> Product1/2
  Product3/1 -> Sum2/2
  Product1/1 -> Sum2/1
  [vdn] -> Product3/1
  Mux3/1 -> Product3/2
  [vqn] -> Product1/1
  Sum2/1 -> Gain1/1
  [iqn] -> Gain3/1, Mux1/1
  [idn] -> Mux3/1, Mux1/2
  vq-/1 -> [vqn]
  vd-/1 -> [vdn]
  iq-/1 -> [iqn]
  id-/1 -> [idn]
  Gain1/1 -> Gain4/1
  Gain4/1 -> Sum1/2

== system Scenario_2_v2/G3/VSC v2/VSC Control/Control loops/Phasor I ref/Outer-loop/Power calculation ==
  note: AC power calculation using symmetrical components in dq axis
  note: Pavgp = 3/2*(vqp*iqp + vdp*idp) and Qavgp = 3/2*(vqp*idp-vdp*iqp)
  note: P = Pavg + Pc2*cos(2wt) + Ps2*sin(2wt) ---> Pavg = Pavgp + Pavgn
  note: Q = Qavg + Qc2*cos(2wt) + Qs2*sin(2wt) ---> Qavg = Qavgp + Qavgn
  note: Pavgn = 3/2*(vqn*iqn + vdn*idn) and Qavgn = 3/2*(vqn*idn-vdn*iqn)
  vq+ : Inport
  vd+ : Inport  Port=2
  iq+ : Inport  Port=3
  id+ : Inport  Port=4
  vq- : Inport  Port=5
  vd- : Inport  Port=6
  iq- : Inport  Port=7
  id- : Inport  Port=8
  Gain : Gain  Gain=3/2
  Gain1 : Gain  Gain=3/2
  Gain2 : Gain  Gain=-1
  Gain3 : Gain  Gain=-1
  Gain4 : Gain  Gain=negseq_en
  Mux{,1..3} (4 alike) : Mux  Inputs=2
  Product{,1..3} (4 alike) : Product
  Sum1 : Sum
  Sum2 : Sum
  Sum8 : Sum
  PQ : Outport
  wires:
  Sum8/1 -> Gain/1
  Gain2/1 -> Mux2/2
  Mux2/1 -> Product2/2
  Product2/1 -> Sum8/2
  Mux/1 -> Product/2
  Product/1 -> Sum8/1
  iq+/1 -> [iqp]
  [iqp] -> Gain2/1, Mux/1
  id+/1 -> [idp]
  [idp] -> Mux2/1, Mux/2
  vq+/1 -> [vqp]
  [vqp] -> Product/1
  vd+/1 -> [vdp]
  [vdp] -> Product2/1
  Gain/1 -> Sum1/1
  Sum1/1 -> PQ/1
  Gain3/1 -> Mux3/2
  Mux1/1 -> Product1/2
  Product3/1 -> Sum2/2
  Product1/1 -> Sum2/1
  [vdn] -> Product3/1
  Mux3/1 -> Product3/2
  [vqn] -> Product1/1
  Sum2/1 -> Gain1/1
  [iqn] -> Gain3/1, Mux1/1
  [idn] -> Mux3/1, Mux1/2
  vq-/1 -> [vqn]
  vd-/1 -> [vdn]
  iq-/1 -> [iqn]
  id-/1 -> [idn]
  Gain1/1 -> Gain4/1
  Gain4/1 -> Sum1/2

== system Scenario_2_v2/G3/VSC v2/VSC Control/Control loops/Phasor PQ 1st/Outer-loop/Power calculation ==
  note: AC power calculation using symmetrical components in dq axis
  note: Pavgp = 3/2*(vqp*iqp + vdp*idp) and Qavgp = 3/2*(vqp*idp-vdp*iqp)
  note: P = Pavg + Pc2*cos(2wt) + Ps2*sin(2wt) ---> Pavg = Pavgp + Pavgn
  note: Q = Qavg + Qc2*cos(2wt) + Qs2*sin(2wt) ---> Qavg = Qavgp + Qavgn
  note: Pavgn = 3/2*(vqn*iqn + vdn*idn) and Qavgn = 3/2*(vqn*idn-vdn*iqn)
  vq+ : Inport
  vd+ : Inport  Port=2
  iq+ : Inport  Port=3
  id+ : Inport  Port=4
  vq- : Inport  Port=5
  vd- : Inport  Port=6
  iq- : Inport  Port=7
  id- : Inport  Port=8
  Gain : Gain  Gain=3/2
  Gain1 : Gain  Gain=3/2
  Gain2 : Gain  Gain=-1
  Gain3 : Gain  Gain=-1
  Gain4 : Gain  Gain=negseq_en
  Mux{,1..3} (4 alike) : Mux  Inputs=2
  Product{,1..3} (4 alike) : Product
  Sum1 : Sum
  Sum2 : Sum
  Sum8 : Sum
  PQ : Outport
  wires:
  Sum8/1 -> Gain/1
  Gain2/1 -> Mux2/2
  Mux2/1 -> Product2/2
  Product2/1 -> Sum8/2
  Mux/1 -> Product/2
  Product/1 -> Sum8/1
  iq+/1 -> [iqp]
  [iqp] -> Gain2/1, Mux/1
  id+/1 -> [idp]
  [idp] -> Mux2/1, Mux/2
  vq+/1 -> [vqp]
  [vqp] -> Product/1
  vd+/1 -> [vdp]
  [vdp] -> Product2/1
  Gain/1 -> Sum1/1
  Sum1/1 -> PQ/1
  Gain3/1 -> Mux3/2
  Mux1/1 -> Product1/2
  Product3/1 -> Sum2/2
  Product1/1 -> Sum2/1
  [vdn] -> Product3/1
  Mux3/1 -> Product3/2
  [vqn] -> Product1/1
  Sum2/1 -> Gain1/1
  [iqn] -> Gain3/1, Mux1/1
  [idn] -> Mux3/1, Mux1/2
  vq-/1 -> [vqn]
  vd-/1 -> [vdn]
  iq-/1 -> [iqn]
  id-/1 -> [idn]
  Gain1/1 -> Gain4/1
  Gain4/1 -> Sum1/2

== system Scenario_2_v2/G3/VSC v2/VSC Control/Control loops/SW, EMT AVG, Phasor Quasi-EMT/Outer-loop/Power calculation ==
  note: AC power calculation using symmetrical components in dq axis
  note: Pavgp = 3/2*(vqp*iqp + vdp*idp) and Qavgp = 3/2*(vqp*idp-vdp*iqp)
  note: P = Pavg + Pc2*cos(2wt) + Ps2*sin(2wt) ---> Pavg = Pavgp + Pavgn
  note: Q = Qavg + Qc2*cos(2wt) + Qs2*sin(2wt) ---> Qavg = Qavgp + Qavgn
  note: Pavgn = 3/2*(vqn*iqn + vdn*idn) and Qavgn = 3/2*(vqn*idn-vdn*iqn)
  vq+ : Inport
  vd+ : Inport  Port=2
  iq+ : Inport  Port=3
  id+ : Inport  Port=4
  vq- : Inport  Port=5
  vd- : Inport  Port=6
  iq- : Inport  Port=7
  id- : Inport  Port=8
  Gain : Gain  Gain=3/2
  Gain1 : Gain  Gain=3/2
  Gain2 : Gain  Gain=-1
  Gain3 : Gain  Gain=-1
  Gain4 : Gain  Gain=negseq_en
  Mux{,1..3} (4 alike) : Mux  Inputs=2
  Product{,1..3} (4 alike) : Product
  Sum1 : Sum
  Sum2 : Sum
  Sum8 : Sum
  PQ : Outport
  wires:
  Sum8/1 -> Gain/1
  Gain2/1 -> Mux2/2
  Mux2/1 -> Product2/2
  Product2/1 -> Sum8/2
  Mux/1 -> Product/2
  Product/1 -> Sum8/1
  iq+/1 -> [iqp]
  [iqp] -> Gain2/1, Mux/1
  id+/1 -> [idp]
  [idp] -> Mux2/1, Mux/2
  vq+/1 -> [vqp]
  [vqp] -> Product/1
  vd+/1 -> [vdp]
  [vdp] -> Product2/1
  Gain/1 -> Sum1/1
  Sum1/1 -> PQ/1
  Gain3/1 -> Mux3/2
  Mux1/1 -> Product1/2
  Product3/1 -> Sum2/2
  Product1/1 -> Sum2/1
  [vdn] -> Product3/1
  Mux3/1 -> Product3/2
  [vqn] -> Product1/1
  Sum2/1 -> Gain1/1
  [iqn] -> Gain3/1, Mux1/1
  [idn] -> Mux3/1, Mux1/2
  vq-/1 -> [vqn]
  vd-/1 -> [vdn]
  iq-/1 -> [iqn]
  id-/1 -> [idn]
  Gain1/1 -> Gain4/1
  Gain4/1 -> Sum1/2

== system Scenario_2_v2/G3/VSC v2/VSC Control/Control loops/SW, EMT AVG, Phasor Quasi-EMT/Outer-loop/Subsystem2 ==
  note: Hold initial variable value for a given time
  In1 : Inport
  Constant : Constant  Value=x0
  Constant1 : Constant
  Integrator : Integrator
  Switch : Switch  Threshold=Td
  Out1 : Outport
  wires:
  Integrator/1 -> Switch/2
  In1/1 -> Switch/1
  Switch/1 -> Out1/1
  Constant/1 -> Switch/3
  Constant1/1 -> Integrator/1

== system Scenario_2_v2/G3/VSC v2/VSC Control/Control loops/SW, EMT AVG, Phasor Quasi-EMT/Outer-loop/Subsystem3 ==
  note: Hold initial variable value for a given time
  In1 : Inport
  Constant : Constant  Value=x0
  Constant1 : Constant
  Integrator : Integrator
  Switch : Switch  Threshold=Td
  Out1 : Outport
  wires:
  Integrator/1 -> Switch/2
  In1/1 -> Switch/1
  Switch/1 -> Out1/1
  Constant/1 -> Switch/3
  Constant1/1 -> Integrator/1

== system Scenario_2_v2/G3/VSC v2/VSC Control/Measurements/EMT/PLL aligned with positive-sequence/Phase-sequence separation ==
  note: Phase-sequence separation based on
      | Delayed Signal Cancellation (DSC) method
  abc : Inport
  Theta : Inport  Port=2
  Complex to Real-Imag1 : ComplexToRealImag
  Complex to Real-Imag2 : ComplexToRealImag
  Complex to Real-Imag3 : ComplexToRealImag
  Constant : Constant  Value=negseq_en
  Demux3 : Demux  Outputs=3
  Exp2 : Math  OutputSignalType=complex  SaturateOnIntegerOverflow=on
  Exp3 : Math  OutputSignalType=complex  SaturateOnIntegerOverflow=on
  Gain1 : Gain  Gain=1/2
  Gain4 : Gain  Gain=-1i
  Gain5 : Gain  Gain=1i
  Gain6 : Gain  Gain=1/2
  Gain7 : Gain  Gain=1i
  NOT : Logic  Operator=NOT  IconShape=distinctive  AllPortsSameDT=off  OutDataTypeStr=boolean
  Product3 : Product
  Product4 : Product
  Real-Imag to Complex : RealImagToComplex
  Real-Imag to Complex1 : RealImagToComplex
  Sum1 : Sum  Inputs=|++
  Sum2 : Sum  Inputs=-+|
  Switch : Switch  Criteria=u2 ~= 0
  Terminator3 : Terminator
  Transport Delay2 : TransportDelay  DelayTime=1/4*(1/fg)  BufferSize=1024*4
  Transport Delay3 : TransportDelay  DelayTime=1/4*(1/fg)  BufferSize=1024*4
  abc to Alpha-Beta-Zero : powerlib_meascontrol/Transformations/abc to Alpha-Beta-Zero
  q+ : Outport
  d+ : Outport  Port=2
  q- : Outport  Port=3
  d- : Outport  Port=4
  wires:
  NOT/1 -> Switch/2
  Constant/1 -> NOT/1
  Switch/1 -> Product3/1
  Gain6/1 -> Switch/3
  Sum2/1 -> Gain1/1
  Transport Delay2/1 -> Real-Imag to Complex1/1
  Demux3/1 -> Real-Imag to Complex/1
  Complex to Real-Imag1/2 -> Transport Delay3/1
  Gain1/1 -> Product4/2
  Real-Imag to Complex/1 -> Complex to Real-Imag1/1, Sum2/2, Sum1/1, Switch/1
  Complex to Real-Imag3/1 -> d-/1
  Real-Imag to Complex1/1 -> Gain5/1
  Complex to Real-Imag1/1 -> Transport Delay2/1
  Transport Delay3/1 -> Real-Imag to Complex1/2
  Demux3/2 -> Real-Imag to Complex/2
  Product3/1 -> Complex to Real-Imag2/1
  Product4/1 -> Complex to Real-Imag3/1
  abc to Alpha-Beta-Zero/1 -> Demux3/1
  abc/1 -> abc to Alpha-Beta-Zero/1
  Exp3/1 -> Product4/1
  Complex to Real-Imag3/2 -> q-/1
  Complex to Real-Imag2/2 -> q+/1
  Demux3/3 -> Terminator3/1
  Sum1/1 -> Gain6/1
  Gain5/1 -> Sum2/1, Sum1/2
  Exp2/1 -> Product3/2
  Gain4/1 -> Exp2/1
  Theta/1 -> Gain4/1, Gain7/1
  Gain7/1 -> Exp3/1
  Complex to Real-Imag2/1 -> d+/1

== system Scenario_2_v2/G3/VSC v2/VSC Control/Measurements/EMT/PLL aligned with positive-sequence/Subsystem ==
  note: PI controller with reset port and initial conditions restored after reset or after maximum/minimum values are reached
  in : Inport
  Reset : Inport  Port=2
  Compare To Constant2 : simulink/Logic and Bit Operations/Compare To Constant  relop=~=  const=0  OutDataTypeStr=boolean
  Constant2 : Constant  Value=2*pi*fg
  Gain : Gain  Gain=kp_pll
  Gain1 : Gain  Gain=kp_pll/tau_pll
  Integrator Limited : Integrator  ExternalReset=level  InitialCondition=2*pi*fg  UpperSaturationLimit=10.1*2*pi*fg  LowerSaturationLimit=0.09*2*pi*fg  ShowSaturationPort=on
  Memory1 : Memory
  NOT : Logic  Operator=NOT  IconShape=distinctive  AllPortsSameDT=off  OutDataTypeStr=boolean
  OR2 : Logic  Operator=OR  IconShape=distinctive  AllPortsSameDT=off  OutDataTypeStr=boolean
  Product : Product
  Sum : Sum
  Switch1 : Switch
  w : Outport
  wires:
  Switch1/1 -> w/1
  Product/1 -> Gain1/1, Gain/1
  Gain1/1 -> Integrator Limited/1
  Integrator Limited/2 -> Compare To Constant2/1, Switch1/2
  Compare To Constant2/1 -> Memory1/1
  OR2/1 -> Integrator Limited/2, NOT/1
  Constant2/1 -> Switch1/3
  Memory1/1 -> OR2/1
  Reset/1 -> OR2/2
  Gain/1 -> Sum/1
  Integrator Limited/1 -> Sum/2
  Sum/1 -> Switch1/1
  in/1 -> Product/1
  NOT/1 -> Product/2

== system Scenario_2_v2/G5/VSC v2/VSC Control/Control loops/Phasor I 1st/Outer-loop/Power calculation ==
  note: AC power calculation using symmetrical components in dq axis
  note: Pavgp = 3/2*(vqp*iqp + vdp*idp) and Qavgp = 3/2*(vqp*idp-vdp*iqp)
  note: P = Pavg + Pc2*cos(2wt) + Ps2*sin(2wt) ---> Pavg = Pavgp + Pavgn
  note: Q = Qavg + Qc2*cos(2wt) + Qs2*sin(2wt) ---> Qavg = Qavgp + Qavgn
  note: Pavgn = 3/2*(vqn*iqn + vdn*idn) and Qavgn = 3/2*(vqn*idn-vdn*iqn)
  vq+ : Inport
  vd+ : Inport  Port=2
  iq+ : Inport  Port=3
  id+ : Inport  Port=4
  vq- : Inport  Port=5
  vd- : Inport  Port=6
  iq- : Inport  Port=7
  id- : Inport  Port=8
  Gain : Gain  Gain=3/2
  Gain1 : Gain  Gain=3/2
  Gain2 : Gain  Gain=-1
  Gain3 : Gain  Gain=-1
  Gain4 : Gain  Gain=negseq_en
  Mux{,1..3} (4 alike) : Mux  Inputs=2
  Product{,1..3} (4 alike) : Product
  Sum1 : Sum
  Sum2 : Sum
  Sum8 : Sum
  PQ : Outport
  wires:
  Sum8/1 -> Gain/1
  Gain2/1 -> Mux2/2
  Mux2/1 -> Product2/2
  Product2/1 -> Sum8/2
  Mux/1 -> Product/2
  Product/1 -> Sum8/1
  iq+/1 -> [iqp]
  [iqp] -> Gain2/1, Mux/1
  id+/1 -> [idp]
  [idp] -> Mux2/1, Mux/2
  vq+/1 -> [vqp]
  [vqp] -> Product/1
  vd+/1 -> [vdp]
  [vdp] -> Product2/1
  Gain/1 -> Sum1/1
  Sum1/1 -> PQ/1
  Gain3/1 -> Mux3/2
  Mux1/1 -> Product1/2
  Product3/1 -> Sum2/2
  Product1/1 -> Sum2/1
  [vdn] -> Product3/1
  Mux3/1 -> Product3/2
  [vqn] -> Product1/1
  Sum2/1 -> Gain1/1
  [iqn] -> Gain3/1, Mux1/1
  [idn] -> Mux3/1, Mux1/2
  vq-/1 -> [vqn]
  vd-/1 -> [vdn]
  iq-/1 -> [iqn]
  id-/1 -> [idn]
  Gain1/1 -> Gain4/1
  Gain4/1 -> Sum1/2

== system Scenario_2_v2/G5/VSC v2/VSC Control/Control loops/Phasor I ref/Outer-loop/Power calculation ==
  note: AC power calculation using symmetrical components in dq axis
  note: Pavgp = 3/2*(vqp*iqp + vdp*idp) and Qavgp = 3/2*(vqp*idp-vdp*iqp)
  note: P = Pavg + Pc2*cos(2wt) + Ps2*sin(2wt) ---> Pavg = Pavgp + Pavgn
  note: Q = Qavg + Qc2*cos(2wt) + Qs2*sin(2wt) ---> Qavg = Qavgp + Qavgn
  note: Pavgn = 3/2*(vqn*iqn + vdn*idn) and Qavgn = 3/2*(vqn*idn-vdn*iqn)
  vq+ : Inport
  vd+ : Inport  Port=2
  iq+ : Inport  Port=3
  id+ : Inport  Port=4
  vq- : Inport  Port=5
  vd- : Inport  Port=6
  iq- : Inport  Port=7
  id- : Inport  Port=8
  Gain : Gain  Gain=3/2
  Gain1 : Gain  Gain=3/2
  Gain2 : Gain  Gain=-1
  Gain3 : Gain  Gain=-1
  Gain4 : Gain  Gain=negseq_en
  Mux{,1..3} (4 alike) : Mux  Inputs=2
  Product{,1..3} (4 alike) : Product
  Sum1 : Sum
  Sum2 : Sum
  Sum8 : Sum
  PQ : Outport
  wires:
  Sum8/1 -> Gain/1
  Gain2/1 -> Mux2/2
  Mux2/1 -> Product2/2
  Product2/1 -> Sum8/2
  Mux/1 -> Product/2
  Product/1 -> Sum8/1
  iq+/1 -> [iqp]
  [iqp] -> Gain2/1, Mux/1
  id+/1 -> [idp]
  [idp] -> Mux2/1, Mux/2
  vq+/1 -> [vqp]
  [vqp] -> Product/1
  vd+/1 -> [vdp]
  [vdp] -> Product2/1
  Gain/1 -> Sum1/1
  Sum1/1 -> PQ/1
  Gain3/1 -> Mux3/2
  Mux1/1 -> Product1/2
  Product3/1 -> Sum2/2
  Product1/1 -> Sum2/1
  [vdn] -> Product3/1
  Mux3/1 -> Product3/2
  [vqn] -> Product1/1
  Sum2/1 -> Gain1/1
  [iqn] -> Gain3/1, Mux1/1
  [idn] -> Mux3/1, Mux1/2
  vq-/1 -> [vqn]
  vd-/1 -> [vdn]
  iq-/1 -> [iqn]
  id-/1 -> [idn]
  Gain1/1 -> Gain4/1
  Gain4/1 -> Sum1/2

== system Scenario_2_v2/G5/VSC v2/VSC Control/Control loops/Phasor PQ 1st/Outer-loop/Power calculation ==
  note: AC power calculation using symmetrical components in dq axis
  note: Pavgp = 3/2*(vqp*iqp + vdp*idp) and Qavgp = 3/2*(vqp*idp-vdp*iqp)
  note: P = Pavg + Pc2*cos(2wt) + Ps2*sin(2wt) ---> Pavg = Pavgp + Pavgn
  note: Q = Qavg + Qc2*cos(2wt) + Qs2*sin(2wt) ---> Qavg = Qavgp + Qavgn
  note: Pavgn = 3/2*(vqn*iqn + vdn*idn) and Qavgn = 3/2*(vqn*idn-vdn*iqn)
  vq+ : Inport
  vd+ : Inport  Port=2
  iq+ : Inport  Port=3
  id+ : Inport  Port=4
  vq- : Inport  Port=5
  vd- : Inport  Port=6
  iq- : Inport  Port=7
  id- : Inport  Port=8
  Gain : Gain  Gain=3/2
  Gain1 : Gain  Gain=3/2
  Gain2 : Gain  Gain=-1
  Gain3 : Gain  Gain=-1
  Gain4 : Gain  Gain=negseq_en
  Mux{,1..3} (4 alike) : Mux  Inputs=2
  Product{,1..3} (4 alike) : Product
  Sum1 : Sum
  Sum2 : Sum
  Sum8 : Sum
  PQ : Outport
  wires:
  Sum8/1 -> Gain/1
  Gain2/1 -> Mux2/2
  Mux2/1 -> Product2/2
  Product2/1 -> Sum8/2
  Mux/1 -> Product/2
  Product/1 -> Sum8/1
  iq+/1 -> [iqp]
  [iqp] -> Gain2/1, Mux/1
  id+/1 -> [idp]
  [idp] -> Mux2/1, Mux/2
  vq+/1 -> [vqp]
  [vqp] -> Product/1
  vd+/1 -> [vdp]
  [vdp] -> Product2/1
  Gain/1 -> Sum1/1
  Sum1/1 -> PQ/1
  Gain3/1 -> Mux3/2
  Mux1/1 -> Product1/2
  Product3/1 -> Sum2/2
  Product1/1 -> Sum2/1
  [vdn] -> Product3/1
  Mux3/1 -> Product3/2
  [vqn] -> Product1/1
  Sum2/1 -> Gain1/1
  [iqn] -> Gain3/1, Mux1/1
  [idn] -> Mux3/1, Mux1/2
  vq-/1 -> [vqn]
  vd-/1 -> [vdn]
  iq-/1 -> [iqn]
  id-/1 -> [idn]
  Gain1/1 -> Gain4/1
  Gain4/1 -> Sum1/2
